simulink model "lab7schema"  (R2023b)
settings: Solver=VariableStepAuto  StartTime=0.0  StopTime=10  RelTol=1e-3
undefined symbols (not defined in the file): d, DiscIntNeverNeededParam, i, p
libraries: checkpacklib x1
settings Model: Creator=user  LastModifiedBy=killer

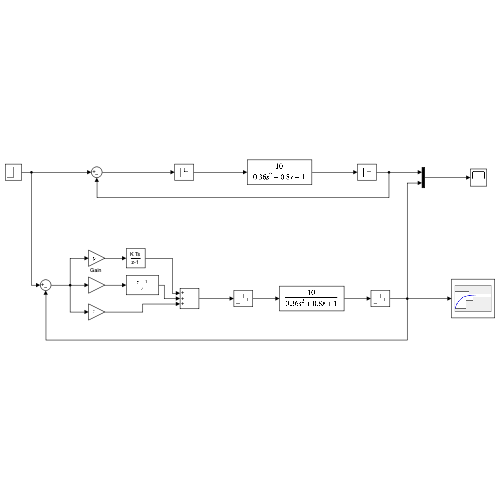
[thumbnail: Simulink's stored preview of the top-level diagram]
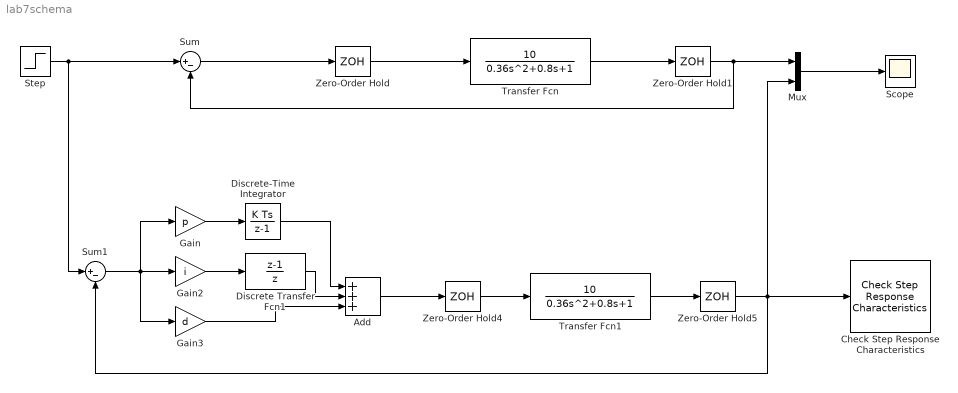
== system lab7schema ==
  Add : Sum  Inputs=+++
  Check Step Response Characteristics : checkpacklib/Check Step Response  Characteristics  InstantiateOnLoad=on  enabled=on  stopWhenAssertionFail=off  export=off  ViewDlgPos=[]  OpenViewOnLoad=off  LaunchViewOnOpen=off  TimeUnits=seconds  EnableStepResponseBound=on  InitialValue=0  FinalValue=1  StepTime=0  RiseTime=5  PercentRise=80  SettlingTime=7  PercentSettling=1  PercentOvershoot=10  PercentUndershoot=1
      settings: LibrarySourceBlock=|
      | sdolib/Model Verification/Check Step Response
      | Characteristics
  Discrete Transfer Fcn1 : DiscreteTransferFcn  Numerator=[1 -1]  Denominator=[1 0]
  Discrete-Time Integrator : DiscreteIntegrator  SampleTime=0.01  ICPrevOutput=DiscIntNeverNeededParam  ICPrevScaledInput=DiscIntNeverNeededParam
  "Gain " : Gain  Gain=p
  Gain2 : Gain  Gain=i
  Gain3 : Gain  Gain=d
  Mux : Mux  Inputs=2
  Scope : Scope
  Step : Step  Time=0  SampleTime=0
  Sum : Sum  Inputs=|+-
  Sum1 : Sum  Inputs=|+-
  Transfer Fcn : TransferFcn  Numerator=[10]  Denominator=[0.36 0.8 1]
  Transfer Fcn1 : TransferFcn  Numerator=[10]  Denominator=[0.36 0.8 1]
  Zero-Order Hold{,1,4..5} (4 alike) : ZeroOrderHold  SampleTime=0.01
  wires:
  Step/1 -> Sum/1, Sum1/1
  Sum/1 -> Zero-Order Hold/1
  Zero-Order Hold/1 -> Transfer Fcn/1
  Transfer Fcn/1 -> Zero-Order Hold1/1
  Zero-Order Hold1/1 -> Sum/2, Mux/1
  Mux/1 -> Scope/1
  Sum1/1 -> Gain3/1, Gain2/1, "Gain "/1
  Add/1 -> Zero-Order Hold4/1
  Zero-Order Hold4/1 -> Transfer Fcn1/1
  Transfer Fcn1/1 -> Zero-Order Hold5/1
  Zero-Order Hold5/1 -> Sum1/2, Mux/2, Check Step Response Characteristics/1
  Gain3/1 -> Add/3
  Gain2/1 -> Discrete Transfer Fcn1/1
  Discrete Transfer Fcn1/1 -> Add/2
  "Gain "/1 -> Discrete-Time Integrator/1
  Discrete-Time Integrator/1 -> Add/1
